simulink model "P6_son"  (R2021b)
settings: Solver=VariableStepAuto  StartTime=0.0  StopTime=10.0  RelTol=1e-3
undefined symbols (not defined in the file or in its folder): A1, b, B1, k11, k12, k21, k22, L, n00, sample_time, v
libraries: simulink x1
settings Model: Creator=11639  LastModifiedBy=11639

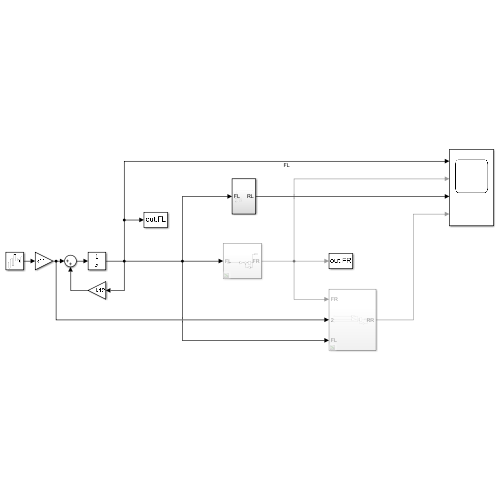
[thumbnail: Simulink's stored preview of the top-level diagram]
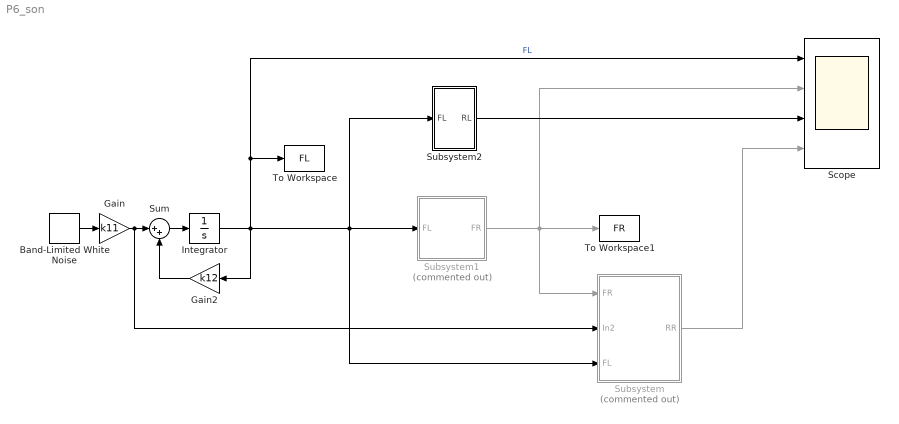
== system P6_son ==
  Band-Limited White Noise : simulink/Sources/Band-Limited White Noise  Cov=noise_power  Ts=sample_time  seed=seed
  Gain : Gain  Gain=k11
  Gain2 : Gain  Gain=k12
  Integrator : Integrator
  Scope : Scope  NumInputPorts=4
  Subsystem : Subsystem  Commented=on
  Subsystem1 : Subsystem  Commented=on
  Subsystem2 : Subsystem
  Sum : Sum  Inputs=|++
  To Workspace : ToWorkspace  VariableName=FL  SaveFormat=Timeseries  SampleTime=-1
  To Workspace1 : ToWorkspace  VariableName=FR  SaveFormat=Timeseries  SampleTime=-1
  wires:
  Band-Limited White Noise/1 -> Gain/1
  Gain/1 -> Subsystem/2(In2), Sum/1
  Sum/1 -> Integrator/1
  Integrator/1 -> Scope/1, To Workspace/1, Gain2/1, Subsystem/3(FL), Subsystem2/1(FL), Subsystem1/1(FL)  "FL"
  Gain2/1 -> Sum/2
  Subsystem/1(RR) -> Scope/4
  Subsystem1/1(FR) -> Scope/2, To Workspace1/1, Subsystem/1(FR)
  Subsystem2/1(RL) -> Scope/3

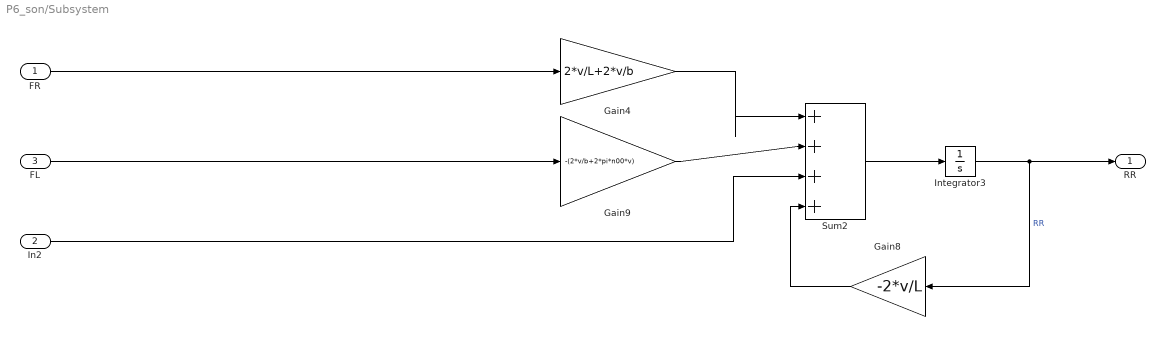
== system P6_son/Subsystem ==
  FR : Inport
  In2 : Inport  Port=2
  FL : Inport  Port=3
  Gain4 : Gain  Gain=2*v/L+2*v/b
  Gain8 : Gain  Gain=-2*v/L
  Gain9 : Gain  Gain=-(2*v/b+2*pi*n00*v)
  Integrator3 : Integrator
  Sum2 : Sum  Inputs=|++++
  RR : Outport
  wires:
  Sum2/1 -> Integrator3/1
  FR/1 -> Gain4/1
  FL/1 -> Gain9/1
  Gain4/1 -> Sum2/1
  Gain9/1 -> Sum2/2
  Integrator3/1 -> RR/1, Gain8/1  "RR"
  In2/1 -> Sum2/3
  Gain8/1 -> Sum2/4

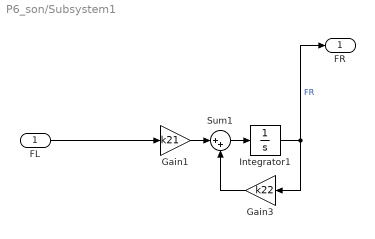
== system P6_son/Subsystem1 ==
  FL : Inport
  Gain1 : Gain  Gain=k21
  Gain3 : Gain  Gain=k22
  Integrator1 : Integrator
  Sum1 : Sum  Inputs=|++
  FR : Outport
  wires:
  Gain3/1 -> Sum1/2
  Integrator1/1 -> FR/1, Gain3/1  "FR"
  Gain1/1 -> Sum1/1
  Sum1/1 -> Integrator1/1
  FL/1 -> Gain1/1

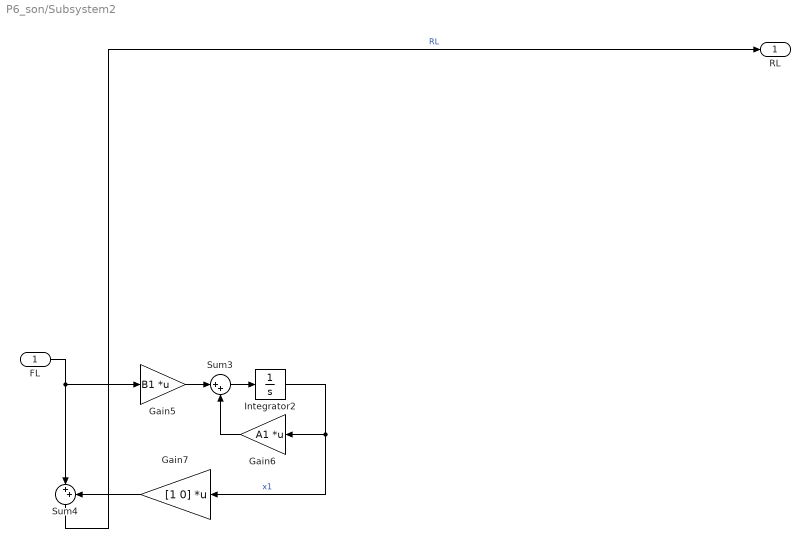
== system P6_son/Subsystem2 ==
  FL : Inport
  Gain5 : Gain  Gain=B1  Multiplication=Matrix(K*u)
  Gain6 : Gain  Gain=A1  Multiplication=Matrix(K*u)
  Gain7 : Gain  Gain=[1 0]  Multiplication=Matrix(K*u)
  Integrator2 : Integrator
  Sum3 : Sum  Inputs=|++
  Sum4 : Sum  Inputs=|++
  RL : Outport
  wires:
  Gain5/1 -> Sum3/1
  FL/1 -> Gain5/1, Sum4/1
  Gain6/1 -> Sum3/2
  Integrator2/1 -> Gain7/1, Gain6/1  "x1"
  Sum3/1 -> Integrator2/1
  Sum4/1 -> RL/1  "RL"
  Gain7/1 -> Sum4/2
